simulink model "mdlref_bus"  (Simulink 6.0)
settings: Solver=ode5  StartTime=0.0  StopTime=30  RelTol=1e-3
PreLoadFcn:
  | load mdlref_counter_bus.mat
settings Model: Creator=The MathWorks Inc.  LastModifiedBy=batserve  ExtModeAutoUpdateStatusClock=off  ProdHWDeviceType=Specified
settings DataIOCC: SignalLoggingName=logsOut
settings OptimizationCC: InlineParams=on
settings DebuggingCC: CheckExecutionContextPreStartOutputMsg=on  CheckExecutionContextRuntimeOutputMsg=on  SolverPrmCheckMsg=none
settings HardwareCC: ProdHWDeviceType=Specified  TargetHWDeviceType=32-bit Generic  ProdEqTarget=off
settings ModelReferenceCC: UpdateModelReferenceTargets=IfOutOfDate
settings RTWCC: GenerateReport=on  ProcessScript=grt_make_rtw_hook  LaunchReport=on

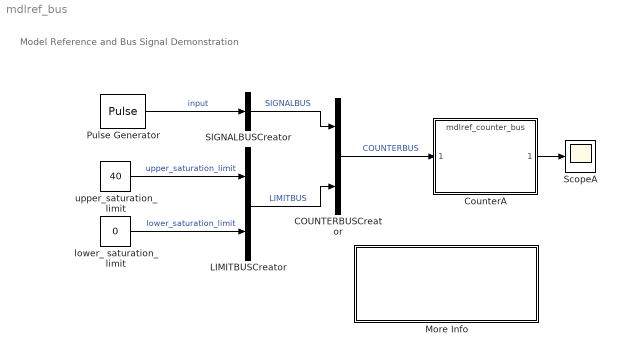
== system mdlref_bus ==
  note: Model Reference and Bus Signal Demonstration
  COUNTERBUSCreator : BusCreator  DialogController=Simulink.DDGSource_Bus  Inputs=2  UseBusObject=on  NonVirtualBus=on
      settings: BusObject=COUNTERBUS
  CounterA : ModelReference  ModelName=mdlref_counter_bus  ModelReferenceVersion=1.111  CopyOfModelName=mdlref_counter_bus
  LIMITBUSCreator : BusCreator  DialogController=Simulink.DDGSource_Bus  Inputs=2  UseBusObject=on  NonVirtualBus=on
      settings: BusObject=LIMITBUS
  More Info : Subsystem  PropExecContextAcrossSSBoundary=on
      settings: OpenFcn=mdlref_busscript
      mask Display: disp('Double click here \nfor a step-by-step\ntutorial on this model')
  Pulse Generator : DiscretePulseGenerator  Amplitude=int32(1)  SampleTime=0.1
  SIGNALBUSCreator : BusCreator  DialogController=Simulink.DDGSource_Bus  Inputs=1  UseBusObject=on  NonVirtualBus=on
      settings: BusObject=SIGNALBUS
  ScopeA : Scope
      settings: TimeRange=30  YMax=50  SaveName=ScopeDataA  DataFormat=Array
  lower_ saturation_ limit : Constant  Value=0  OutDataTypeMode=int32
  upper_saturation_limit : Constant  Value=40  OutDataTypeMode=int32
  wires:
  upper_saturation_limit/1 -> LIMITBUSCreator/1  "upper_saturation_limit"
  lower_ saturation_ limit/1 -> LIMITBUSCreator/2  "lower_saturation_limit"
  LIMITBUSCreator/1 -> COUNTERBUSCreator/2  "LIMITBUS"
  Pulse Generator/1 -> SIGNALBUSCreator/1  "input"
  COUNTERBUSCreator/1 -> CounterA/1  "COUNTERBUS"
  CounterA/1 -> ScopeA/1
  SIGNALBUSCreator/1 -> COUNTERBUSCreator/1  "SIGNALBUS"

== system mdlref_bus/More Info ==
  note: This demonstration shows how signals may be grouped and ungrouped while
      | retaining their names.  In this demonstration, 5 signals are created and labelled
      | appropriately.  These signals are then mux'd together to create a bus of signals.
      | This bus of signals is then fed into the Bus Selector block.  Inside of the Bus
      | Selector block, the Pulse and Chirp signals are chosen to be output from the
      | original signal bus.
      |
      | It is possible to place a nest signal buses and then still retrieve the original signal
      | with its label.
  note: Bus Block Demonstration
